simulink model "MPC_design_model"  (R2023b)
settings: Solver=VariableStepAuto  StartTime=0.0  StopTime=10.0  RelTol=1e-3
values from neighbouring files (symbols this model uses):
  C = [1 0]    [MPC_design.m]    (also in algebraic_design.m = zpk(tf(S, R, Ts)); qp_ip.m = -A; quiz1.m = 1.5 * (z-0.7) / (z-0.9); quiz2.m = 0.4 * (z-0.4) / (z-0.2))
  md = struct('Ps',[], 	    'Ga',[], 	    'Th',[], 	    'Ps_c',[], 	    'Ga_c',[], 	    'Th_c',[], 	    'Qq',[], 	    'Rr',[], 	    'H',[], 	    'F_con',[], 	    'f_con',[], 	    'Gam_con',[], 	    'gam_con',[], 	    'W_con',[], 	    'w_con',[], 	    'K',[], 	    'Kmpc',[], 	    'Ks',[], 	    'Ade',[], 	    'Bde',[], 	    'Cyde',[], 	    'Czde',[], 	    'Dzde',[], 	    'Ccde',[], 	    'Dcde',[], 	    'n' ...(+217 chars)    [MPCInit.m]    (also in MPC_design.m = MPCInit(Ad, Bd, Cy, Cz, Dz, Cc, Dc, Hp, Hw, zblk, Hc, ublk, )
  Ts = 50e-3    (= 0.05)    [MPC_design.m]    (also in algebraic_design.m = 0.002; quiz1.m = 1; quiz2.m = 1; quiz3.m = 0.002)
libraries: cstblocks x1
settings Model: Creator=lucap  LastModifiedBy=lucap

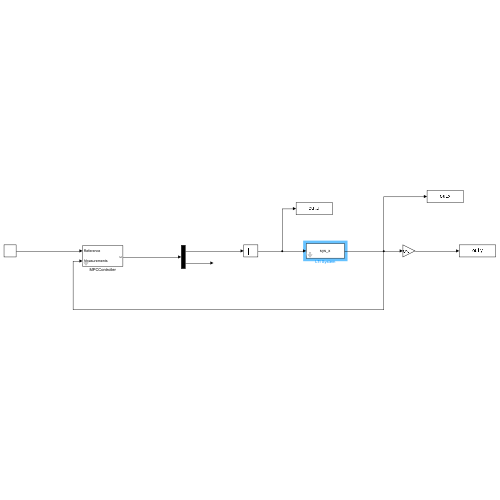
[thumbnail: Simulink's stored preview of the top-level diagram]
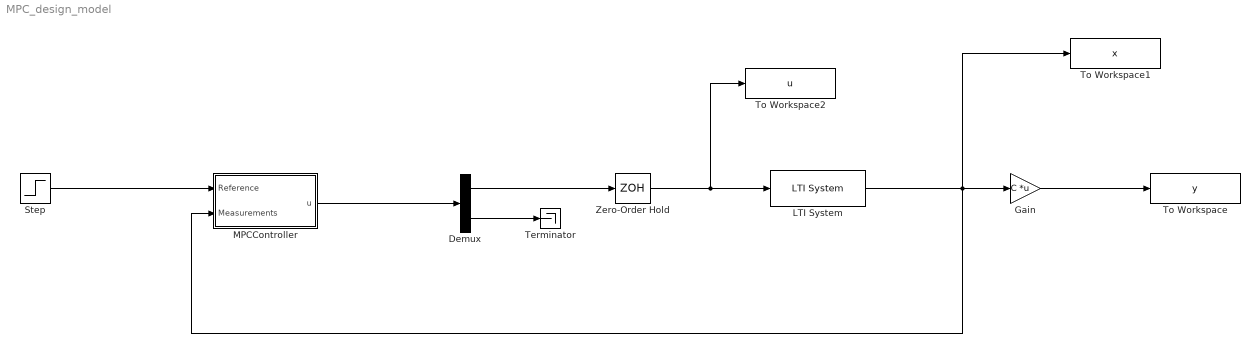
== system MPC_design_model ==
  Demux : Demux  Outputs=2
  Gain : Gain  Gain=C  Multiplication=Matrix(K*u)
  LTI System : cstblocks/LTI System  sys=sys_x  IC=x0  PadeOrder=0
  MPCController : Subsystem  mask{md=md}
      mask prompts: md "MPCData"
  Step : Step  Time=0  SampleTime=0
  Terminator : Terminator
  To Workspace : ToWorkspace  VariableName=y  SaveFormat=Timeseries  SampleTime=Ts * 0.001
  To Workspace1 : ToWorkspace  VariableName=x  SaveFormat=Timeseries  SampleTime=Ts * 0.001
  To Workspace2 : ToWorkspace  VariableName=u  SaveFormat=Timeseries  SampleTime=Ts * 0.001
  Zero-Order Hold : ZeroOrderHold  SampleTime=-1
  wires:
  Step/1 -> MPCController/1(Reference)
  MPCController/1(u) -> Demux/1
  Demux/2 -> Terminator/1
  Demux/1 -> Zero-Order Hold/1
  Zero-Order Hold/1 -> To Workspace2/1, LTI System/1
  LTI System/1 -> To Workspace1/1, MPCController/2(Measurements), Gain/1
  Gain/1 -> To Workspace/1

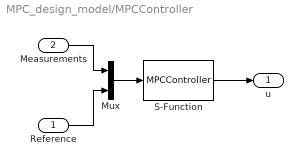
== system MPC_design_model/MPCController ==
  Reference : Inport
  Measurements : Inport  Port=2
  Mux : Mux  Inputs=2
  S-Function : S-Function  FunctionName=MPCController  Parameters=md  SFunctionDeploymentMode=off  EnableBusSupport=off
  u : Outport
  wires:
  Mux/1 -> S-Function/1
  Measurements/1 -> Mux/1
  Reference/1 -> Mux/2
  S-Function/1 -> u/1
